simulink model "adcs_simulator"  (R2018a)
settings: Solver=ode4  StartTime=0  StopTime=10.0  FixedStep=ConfParam.confOrbit.dt  RelTol=1e-3
undefined symbols (not defined in the file): ConfParam
libraries: Command x1, Date x1, Orbit x1, Estimator x1, BdotController x1, IGRF x1, SunEphemeris_MathWorks x1, MTB x1, Magnetometer x1, AeroTorqueA x1, ChangeFrame x1, Qinverse x1
settings Model: Creator=Cédric  LastModifiedBy=Cédric
settings DataIOCC: SaveTime=off
settings DebuggingCC: MultiTaskRateTransMsg=warning

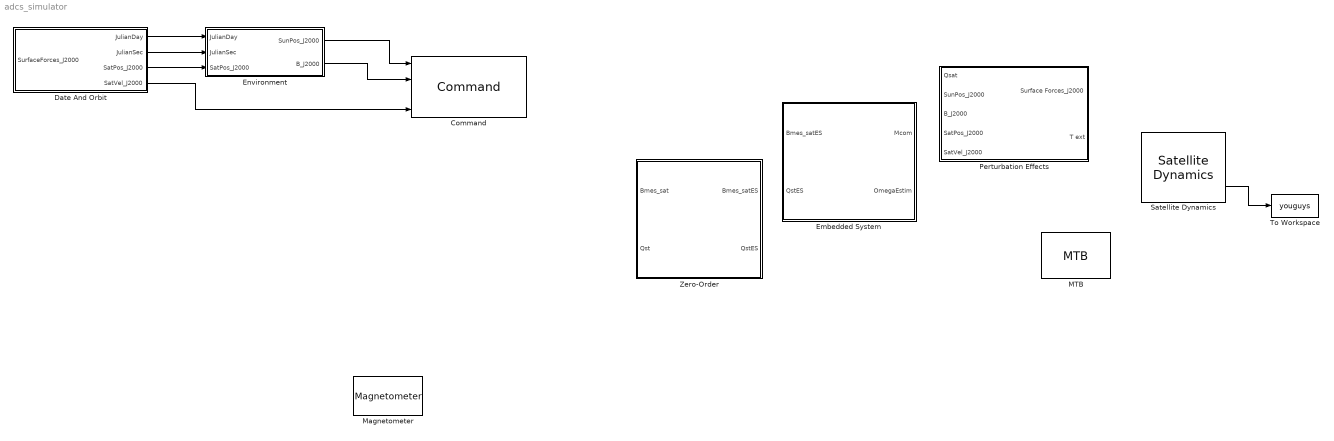
== system adcs_simulator ==
  Command : Command/Command
  Date And Orbit : Subsystem
  Embedded System : Subsystem
  Environment : Subsystem
  MTB : MTB/MTB
  Magnetometer : Magnetometer/Magnetometer
  Perturbation Effects : Subsystem
  Satellite Dynamics : SatDyn/Satellite Dynamics
  To Workspace : ToWorkspace  VariableName=youguys  SaveFormat=Timeseries  SampleTime=-1
  Zero-Order : Subsystem
  wires:
  Date And Orbit/1(JulianDay) -> Environment/1(JulianDay)
  Date And Orbit/2(JulianSec) -> Environment/2(JulianSec)
  Date And Orbit/3(SatPos_J2000) -> Environment/3(SatPos_J2000)
  Environment/2(B_J2000) -> Command/2
  Environment/1(SunPos_J2000) -> Command/1
  Date And Orbit/4(SatVel_J2000) -> Command/4
  Satellite Dynamics/2 -> To Workspace/1

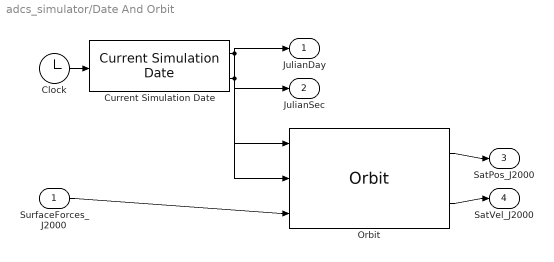
== system adcs_simulator/Date And Orbit ==
  SurfaceForces_J2000 : Inport
  Clock : Clock
  Current Simulation Date : Date/Current Simulation Date
  Orbit : Orbit/Orbit
  JulianDay : Outport
  JulianSec : Outport  Port=2
  SatPos_J2000 : Outport  Port=3
  SatVel_J2000 : Outport  Port=4
  wires:
  Current Simulation Date/1 -> JulianDay/1, Orbit/1
  Current Simulation Date/2 -> JulianSec/1, Orbit/2
  Clock/1 -> Current Simulation Date/1
  SurfaceForces_J2000/1 -> Orbit/3
  Orbit/1 -> SatPos_J2000/1
  Orbit/2 -> SatVel_J2000/1

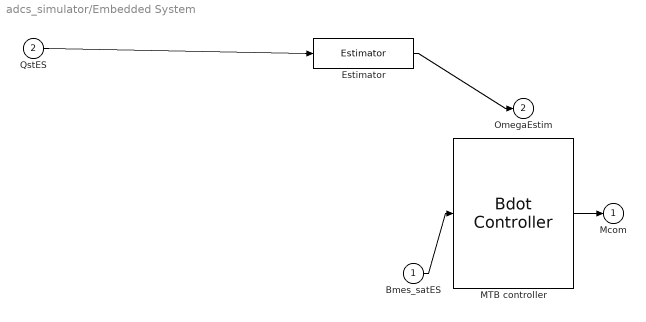
== system adcs_simulator/Embedded System ==
  Bmes_satES : Inport
  QstES : Inport  Port=2
  Estimator : Estimator/Estimator
  MTB controller : BdotController/Bdot Controller
  Mcom : Outport
  OmegaEstim : Outport  Port=2
  wires:
  QstES/1 -> Estimator/1
  Estimator/1 -> OmegaEstim/1
  Bmes_satES/1 -> MTB controller/1
  MTB controller/1 -> Mcom/1

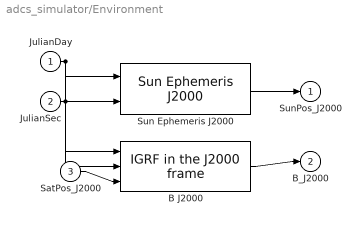
== system adcs_simulator/Environment ==
  JulianDay : Inport
  JulianSec : Inport  Port=2
  SatPos_J2000 : Inport  Port=3
  B J2000 : IGRF/IGRF in the J2000 frame
  Sun Ephemeris J2000 : SunEphemeris_MathWorks/Sun Ephemeris J2000
  SunPos_J2000 : Outport
  B_J2000 : Outport  Port=2
  wires:
  Sun Ephemeris J2000/1 -> SunPos_J2000/1
  JulianDay/1 -> Sun Ephemeris J2000/1, B J2000/1
  JulianSec/1 -> Sun Ephemeris J2000/2, B J2000/2
  SatPos_J2000/1 -> B J2000/3
  B J2000/1 -> B_J2000/1

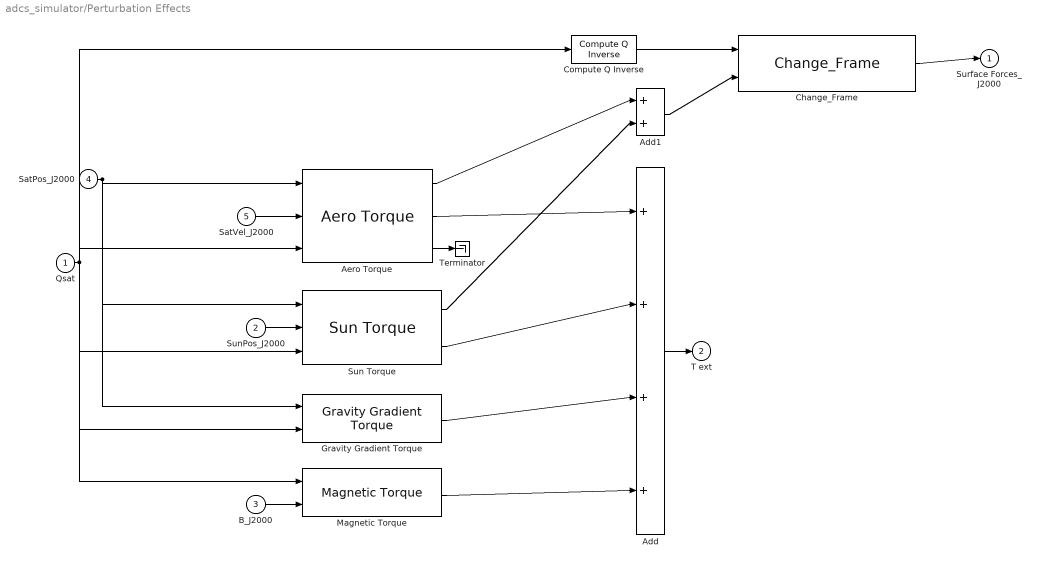
== system adcs_simulator/Perturbation Effects ==
  Qsat : Inport
  SunPos_J2000 : Inport  Port=2
  B_J2000 : Inport  Port=3
  SatPos_J2000 : Inport  Port=4
  SatVel_J2000 : Inport  Port=5
  Add : Sum  Inputs=++++
  Add1 : Sum
  Aero Torque : AeroTorqueA/Aero Torque
  Change_Frame : ChangeFrame/Change_Frame
  Compute Q Inverse : Qinverse/Compute Q Inverse
  Gravity Gradient Torque : GravGradTorque/Gravity Gradient Torque
  Magnetic Torque : MagnTorque/Magnetic Torque
  Sun Torque : SunTorqueA/Sun Torque
  Terminator : Terminator
  Surface Forces_J2000 : Outport
  T ext : Outport  Port=2
  wires:
  Compute Q Inverse/1 -> Change_Frame/1
  Change_Frame/1 -> Surface Forces_J2000/1
  Qsat/1 -> Compute Q Inverse/1, Gravity Gradient Torque/2, Sun Torque/3, Magnetic Torque/1, Aero Torque/3
  SunPos_J2000/1 -> Sun Torque/2
  B_J2000/1 -> Magnetic Torque/2
  SatPos_J2000/1 -> Sun Torque/1, Gravity Gradient Torque/1, Aero Torque/1
  SatVel_J2000/1 -> Aero Torque/2
  Aero Torque/3 -> Terminator/1
  Add1/1 -> Change_Frame/2
  Aero Torque/1 -> Add1/1
  Sun Torque/1 -> Add1/2
  Add/1 -> T ext/1
  Aero Torque/2 -> Add/1
  Sun Torque/2 -> Add/2
  Gravity Gradient Torque/1 -> Add/3
  Magnetic Torque/1 -> Add/4

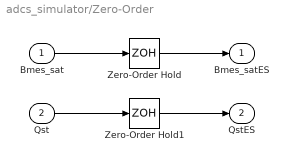
== system adcs_simulator/Zero-Order ==
  Bmes_sat : Inport
  Qst : Inport  Port=2
  Zero-Order Hold : ZeroOrderHold  SampleTime=1/ConfParam.confES.frequency
  Zero-Order Hold1 : ZeroOrderHold  SampleTime=1/ConfParam.confES.frequency
  Bmes_satES : Outport
  QstES : Outport  Port=2
  wires:
  Bmes_sat/1 -> Zero-Order Hold/1
  Zero-Order Hold/1 -> Bmes_satES/1
  Qst/1 -> Zero-Order Hold1/1
  Zero-Order Hold1/1 -> QstES/1
